simulink model "FlatEarth_ports_MATLAB7"  (Simulink 6.2)
settings: Solver=ode45  StartTime=0.0  StopTime=10.0  RelTol=1e-3
undefined symbols (not defined in the file or in its folder): constant, Xa, xIC
settings Model: Creator=andrisan  LastModifiedBy=andrisan  ExtModeAutoUpdateStatusClock=off
settings DataIOCC: SignalLoggingName=sigsOut
settings OptimizationCC: BooleanDataType=off
settings HardwareCC: TargetUnknown=on

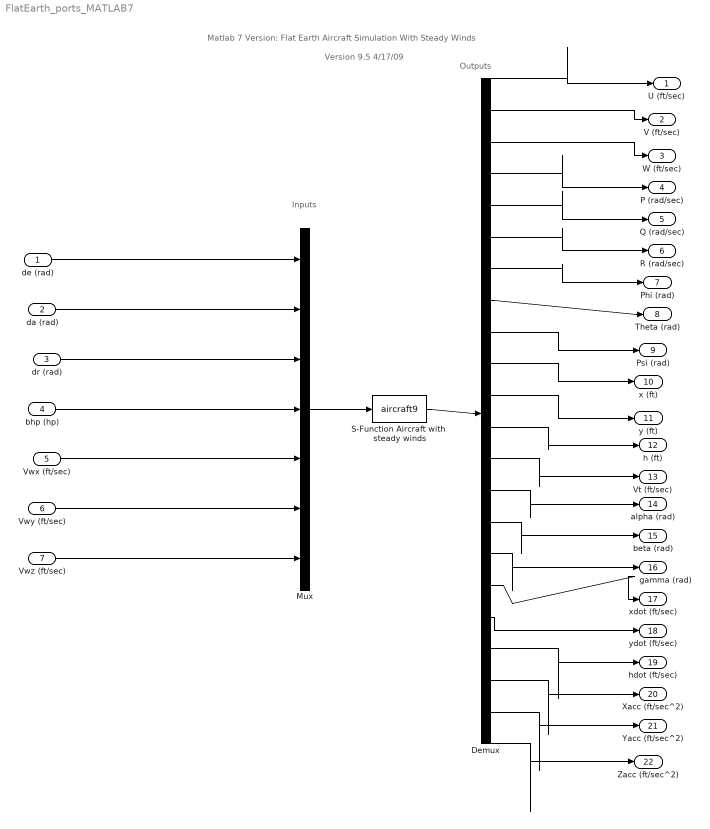
== system FlatEarth_ports_MATLAB7 ==
  note: Matlab 7 Version: Flat Earth Aircraft Simulation With Steady Winds
  note: Version 9.5 4/17/09
  note: Inputs
  note: Outputs
  de (rad) : Inport  Port=1  LatchInput=off
  da (rad) : Inport  Port=2  LatchInput=off
  dr (rad) : Inport  Port=3  LatchInput=off
  bhp (hp) : Inport  Port=4  LatchInput=off
  Vwx (ft/sec) : Inport  Port=5  LatchInput=off
  Vwy (ft/sec) : Inport  Port=6  LatchInput=off
  Vwz (ft/sec) : Inport  Port=7  LatchInput=off
  Demux : Demux  Outputs=22
  Mux : Mux  Inputs=7
  S-Function Aircraft with  steady winds : S-Function  FunctionName=aircraft9  Parameters=constant,xIC,Xa
  U (ft/sec) : Outport
  V (ft/sec) : Outport  Port=2
  W (ft/sec) : Outport  Port=3
  P (rad/sec) : Outport  Port=4
  Q (rad/sec) : Outport  Port=5
  R (rad/sec) : Outport  Port=6
  Phi (rad) : Outport  Port=7
  Theta (rad) : Outport  Port=8
  Psi (rad) : Outport  Port=9
  x (ft) : Outport  Port=10
  y (ft) : Outport  Port=11
  h (ft) : Outport  Port=12
  Vt (ft/sec) : Outport  Port=13
  alpha (rad) : Outport  Port=14
  beta (rad) : Outport  Port=15
  gamma (rad) : Outport  Port=16
  xdot (ft/sec) : Outport  Port=17
  ydot (ft/sec) : Outport  Port=18
  hdot (ft/sec) : Outport  Port=19
  Xacc (ft/sec^2) : Outport  Port=20
  Yacc (ft/sec^2) : Outport  Port=21
  Zacc (ft/sec^2) : Outport  Port=22
  wires:
  S-Function Aircraft with  steady winds/1 -> Demux/1
  Mux/1 -> S-Function Aircraft with  steady winds/1
  de (rad)/1 -> Mux/1
  bhp (hp)/1 -> Mux/4
  Vwx (ft/sec)/1 -> Mux/5
  Vwy (ft/sec)/1 -> Mux/6
  Vwz (ft/sec)/1 -> Mux/7
  dr (rad)/1 -> Mux/3
  da (rad)/1 -> Mux/2
  Demux/1 -> U (ft/sec)/1
  Demux/2 -> V (ft/sec)/1
  Demux/3 -> W (ft/sec)/1
  Demux/4 -> P (rad/sec)/1
  Demux/5 -> Q (rad/sec)/1
  Demux/6 -> R (rad/sec)/1
  Demux/7 -> Phi (rad)/1
  Demux/8 -> Theta (rad)/1
  Demux/9 -> Psi (rad)/1
  Demux/10 -> x (ft)/1
  Demux/11 -> y (ft)/1
  Demux/12 -> h (ft)/1
  Demux/13 -> Vt (ft/sec)/1
  Demux/14 -> alpha (rad)/1
  Demux/15 -> beta (rad)/1
  Demux/16 -> gamma (rad)/1
  Demux/17 -> xdot (ft/sec)/1
  Demux/18 -> ydot (ft/sec)/1
  Demux/19 -> hdot (ft/sec)/1
  Demux/20 -> Xacc (ft/sec^2)/1
  Demux/21 -> Yacc (ft/sec^2)/1
  Demux/22 -> Zacc (ft/sec^2)/1
